simulink model "Examp1"  (Simulink 8.3)
settings: Solver=ode45  StartTime=0.0  StopTime=20.0  RelTol=1e-3
settings Model: Creator=lgw  LastModifiedBy=李广文
settings DataIOCC: SignalLoggingName=sigsOut
settings OptimizationCC: InitFltsAndDblsToZero=on
settings DebuggingCC: SaveWithParameterizedLinksMsg=none  SignalResolutionControl=TryResolveAllWithWarning  SolverPrmCheckMsg=none  MultiTaskDSMMsg=warning  MultiTaskCondExecSysMsg=none  FcnCallInpInsideContextMsg=UseLocalSettings  StateNameClashWarn=none
settings HardwareCC: TargetUnknown=on
settings RTWCC: IncludeERTFirstTime=on
settings GRTTargetCC: TargetFcnLib=ansi_tfl_tmw.mat

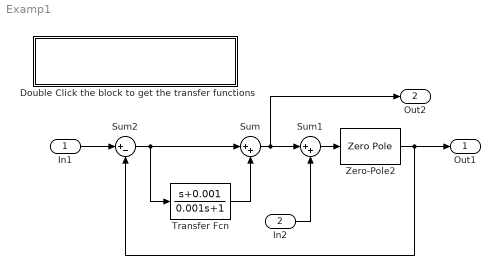
== system Examp1 ==
  In1 : Inport
  In2 : Inport  Port=2
  Double Click the block to get the transfer functions : Subsystem  Description=text('Double Click to get the transfer function')
      settings: OpenFcn=|
      | clc;
      | clear;
      | [A,B,C,D]=linmod('Examp1');
      | G=ss(A,B,C,D);
      | G=tf(G);
      | helpdlg('请到命令窗口观察结果！想想我是怎么做到的？想知道吗？且听下回分解','')
      | disp('所求的传递函数如下所示：')
      | minreal(zpk(G))
  Sum : Sum  Inputs=|++
  Sum1 : Sum  Inputs=|++
  Sum2 : Sum  Inputs=|+-  SaturateOnIntegerOverflow=on
  Transfer Fcn : TransferFcn  Numerator=[1 0.001]  Denominator=[0.001 1]
  Zero-Pole2 : ZeroPole  Zeros=[]  Poles=[ -0.5]
  Out1 : Outport
  Out2 : Outport  Port=2
  wires:
  In1/1 -> Sum2/1
  Zero-Pole2/1 -> Sum2/2, Out1/1
  Sum2/1 -> Transfer Fcn/1, Sum/1
  Transfer Fcn/1 -> Sum/2
  Sum/1 -> Out2/1, Sum1/1
  Sum1/1 -> Zero-Pole2/1
  In2/1 -> Sum1/2

== system Examp1/Double Click the block to get the transfer functions ==
